simulink model "TST_CrCtl_Governor"  (R2016b)
settings: Solver=FixedStepDiscrete  StartTime=0.0  StopTime=simTime  FixedStep=sampleTime  RelTol=1e-3
values from neighbouring files (symbols this model uses):
  testCase = 1    [initTST_CrCtl_Governor_001.m]    (also in initTST_CrCtl_Governor_002.m = 2; initTST_CrCtl_Governor_003.m = 3; initTST_CrCtl_Governor_004.m = 4; initTST_CrCtl_Governor_005.m = 5)
libraries: simulink x144, UnitTest_Lib x110
(part 2 of 7)

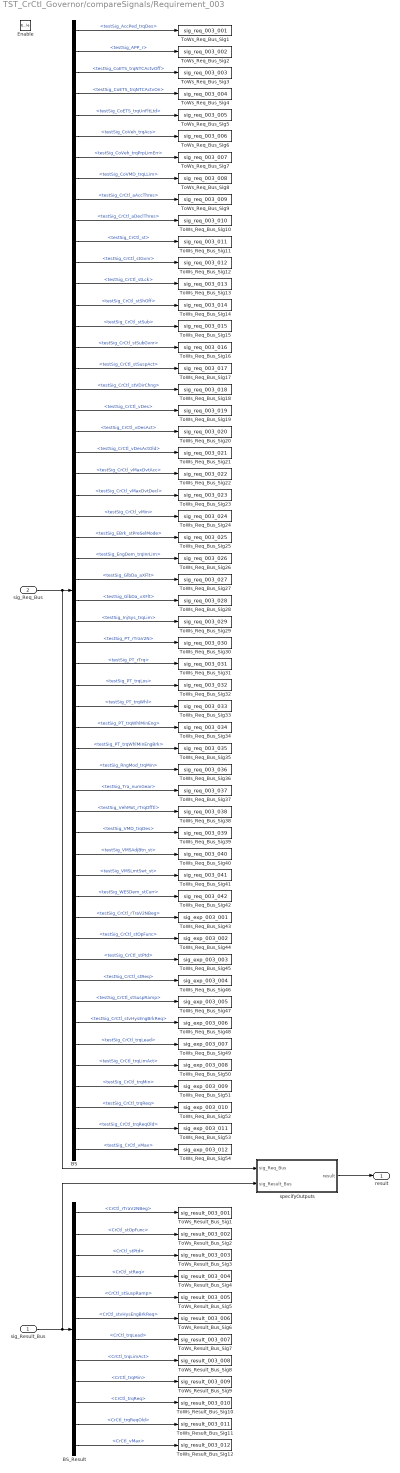
== system TST_CrCtl_Governor/compareSignals/Requirement_003 ==
  sig_Result_Bus : Inport
  sig_Req_Bus : Inport  Port=2
  Enable : EnablePort
  BS : BusSelector  OutputSignals=testSig_AccPed_trqDes,testSig_APP_r,testSig_CoETS_trqNTCActvOff,testSig_CoETS_trqNTCActvOn,testSig_CoETS_trqUnFltLtd,testSig_CoVeh_trqAcs,testSig_CoVeh_trqPrpLimErr,testSig_CoVMD_trqLLim,testSig_CrCtl_aAccThres,testSig_CrCtl_aDeclThres,testSig_CrCtl_st,testSig_CrCtl_stGvnr,testSig_CrCtl_stLck,testSig_CrCtl_stShOff,testSig_CrCtl_stSub,testSig_CrCtl_stSubGvnr,testSig_CrCtl_stSuspAct,testSig_CrCtl_stVDirChng,testSig_CrCtl_vDes,testSig_CrCtl_vDesAct,testSig_CrCtl_vDesActOld,testSig_CrCtl_vMaxDvtAcc,testSig_CrCtl_vMaxDvtDecl,testSig_CrCtl_vMin,testSig_EBrk_stPreSelMode,testSig_EngDem_trqInrLim,testSig_GlbDa_aXFlt,testSig_GlbDa_vXFlt,testSig_InjSys_trqLim,testSig_PT_rTraV2N,testSig_PT_rTrq,testSig_PT_trqLos,testSig_PT_trqWhl,testSig_PT_trqWhlMinEng,testSig_PT_trqWhlMinEngBrk,testSig_RngMod_trqMin,testSig_Tra_numGear,testSig_VehMot_rTrqDfftl,testSig_VMD_trqDes,testSig_VMSAdjBtn_st,testSig_VMSLmtSwt_st,testSig_WESDem_stCurr,testSig_CrCtl_rTraV2NBeg,testSig_CrCtl_stOpFunc,testSig_CrCtl_stPtd,testSig_CrCtl_stReq,testSig_CrCtl_stSuspRamp,testSig_CrCtl_stvHysEngBrkReq,testSig_CrCtl_trqLead,testSig_CrCtl_trqLimAct,testSig_CrCtl_trqMin,testSig_CrCtl_trqReq,testSig_CrCtl_trqReqOld,testSig_CrCtl_vMax
  BS_Result : BusSelector  OutputSignals=CrCtl_rTraV2NBeg,CrCtl_stOpFunc,CrCtl_stPtd,CrCtl_stReq,CrCtl_stSuspRamp,CrCtl_stvHysEngBrkReq,CrCtl_trqLead,CrCtl_trqLimAct,CrCtl_trqMin,CrCtl_trqReq,CrCtl_trqReqOld,CrCtl_vMax
  ToWs_Req_Bus_Sig1 : ToWorkspace  VariableName=sig_req_003_001  SaveFormat=Structure With Time
  ToWs_Req_Bus_Sig10 : ToWorkspace  VariableName=sig_req_003_010  SaveFormat=Structure With Time
  ToWs_Req_Bus_Sig11 : ToWorkspace  VariableName=sig_req_003_011  SaveFormat=Structure With Time
  ToWs_Req_Bus_Sig12 : ToWorkspace  VariableName=sig_req_003_012  SaveFormat=Structure With Time
  ToWs_Req_Bus_Sig13 : ToWorkspace  VariableName=sig_req_003_013  SaveFormat=Structure With Time
  ToWs_Req_Bus_Sig14 : ToWorkspace  VariableName=sig_req_003_014  SaveFormat=Structure With Time
  ToWs_Req_Bus_Sig15 : ToWorkspace  VariableName=sig_req_003_015  SaveFormat=Structure With Time
  ToWs_Req_Bus_Sig16 : ToWorkspace  VariableName=sig_req_003_016  SaveFormat=Structure With Time
  ToWs_Req_Bus_Sig17 : ToWorkspace  VariableName=sig_req_003_017  SaveFormat=Structure With Time
  ToWs_Req_Bus_Sig18 : ToWorkspace  VariableName=sig_req_003_018  SaveFormat=Structure With Time
  ToWs_Req_Bus_Sig19 : ToWorkspace  VariableName=sig_req_003_019  SaveFormat=Structure With Time
  ToWs_Req_Bus_Sig2 : ToWorkspace  VariableName=sig_req_003_002  SaveFormat=Structure With Time
  ToWs_Req_Bus_Sig20 : ToWorkspace  VariableName=sig_req_003_020  SaveFormat=Structure With Time
  ToWs_Req_Bus_Sig21 : ToWorkspace  VariableName=sig_req_003_021  SaveFormat=Structure With Time
  ToWs_Req_Bus_Sig22 : ToWorkspace  VariableName=sig_req_003_022  SaveFormat=Structure With Time
  ToWs_Req_Bus_Sig23 : ToWorkspace  VariableName=sig_req_003_023  SaveFormat=Structure With Time
  ToWs_Req_Bus_Sig24 : ToWorkspace  VariableName=sig_req_003_024  SaveFormat=Structure With Time
  ToWs_Req_Bus_Sig25 : ToWorkspace  VariableName=sig_req_003_025  SaveFormat=Structure With Time
  ToWs_Req_Bus_Sig26 : ToWorkspace  VariableName=sig_req_003_026  SaveFormat=Structure With Time
  ToWs_Req_Bus_Sig27 : ToWorkspace  VariableName=sig_req_003_027  SaveFormat=Structure With Time
  ToWs_Req_Bus_Sig28 : ToWorkspace  VariableName=sig_req_003_028  SaveFormat=Structure With Time
  ToWs_Req_Bus_Sig29 : ToWorkspace  VariableName=sig_req_003_029  SaveFormat=Structure With Time
  ToWs_Req_Bus_Sig3 : ToWorkspace  VariableName=sig_req_003_003  SaveFormat=Structure With Time
  ToWs_Req_Bus_Sig30 : ToWorkspace  VariableName=sig_req_003_030  SaveFormat=Structure With Time
  ToWs_Req_Bus_Sig31 : ToWorkspace  VariableName=sig_req_003_031  SaveFormat=Structure With Time
  ToWs_Req_Bus_Sig32 : ToWorkspace  VariableName=sig_req_003_032  SaveFormat=Structure With Time
  ToWs_Req_Bus_Sig33 : ToWorkspace  VariableName=sig_req_003_033  SaveFormat=Structure With Time
  ToWs_Req_Bus_Sig34 : ToWorkspace  VariableName=sig_req_003_034  SaveFormat=Structure With Time
  ToWs_Req_Bus_Sig35 : ToWorkspace  VariableName=sig_req_003_035  SaveFormat=Structure With Time
  ToWs_Req_Bus_Sig36 : ToWorkspace  VariableName=sig_req_003_036  SaveFormat=Structure With Time
  ToWs_Req_Bus_Sig37 : ToWorkspace  VariableName=sig_req_003_037  SaveFormat=Structure With Time
  ToWs_Req_Bus_Sig38 : ToWorkspace  VariableName=sig_req_003_038  SaveFormat=Structure With Time
  ToWs_Req_Bus_Sig39 : ToWorkspace  VariableName=sig_req_003_039  SaveFormat=Structure With Time
  ToWs_Req_Bus_Sig4 : ToWorkspace  VariableName=sig_req_003_004  SaveFormat=Structure With Time
  ToWs_Req_Bus_Sig40 : ToWorkspace  VariableName=sig_req_003_040  SaveFormat=Structure With Time
  ToWs_Req_Bus_Sig41 : ToWorkspace  VariableName=sig_req_003_041  SaveFormat=Structure With Time
  ToWs_Req_Bus_Sig42 : ToWorkspace  VariableName=sig_req_003_042  SaveFormat=Structure With Time
  ToWs_Req_Bus_Sig43 : ToWorkspace  VariableName=sig_exp_003_001  SaveFormat=Structure With Time
  ToWs_Req_Bus_Sig44 : ToWorkspace  VariableName=sig_exp_003_002  SaveFormat=Structure With Time
  ToWs_Req_Bus_Sig45 : ToWorkspace  VariableName=sig_exp_003_003  SaveFormat=Structure With Time
  ToWs_Req_Bus_Sig46 : ToWorkspace  VariableName=sig_exp_003_004  SaveFormat=Structure With Time
  ToWs_Req_Bus_Sig47 : ToWorkspace  VariableName=sig_exp_003_005  SaveFormat=Structure With Time
  ToWs_Req_Bus_Sig48 : ToWorkspace  VariableName=sig_exp_003_006  SaveFormat=Structure With Time
  ToWs_Req_Bus_Sig49 : ToWorkspace  VariableName=sig_exp_003_007  SaveFormat=Structure With Time
  ToWs_Req_Bus_Sig5 : ToWorkspace  VariableName=sig_req_003_005  SaveFormat=Structure With Time
  ToWs_Req_Bus_Sig50 : ToWorkspace  VariableName=sig_exp_003_008  SaveFormat=Structure With Time
  ToWs_Req_Bus_Sig51 : ToWorkspace  VariableName=sig_exp_003_009  SaveFormat=Structure With Time
  ToWs_Req_Bus_Sig52 : ToWorkspace  VariableName=sig_exp_003_010  SaveFormat=Structure With Time
  ToWs_Req_Bus_Sig53 : ToWorkspace  VariableName=sig_exp_003_011  SaveFormat=Structure With Time
  ToWs_Req_Bus_Sig54 : ToWorkspace  VariableName=sig_exp_003_012  SaveFormat=Structure With Time
  ToWs_Req_Bus_Sig6 : ToWorkspace  VariableName=sig_req_003_006  SaveFormat=Structure With Time
  ToWs_Req_Bus_Sig7 : ToWorkspace  VariableName=sig_req_003_007  SaveFormat=Structure With Time
  ToWs_Req_Bus_Sig8 : ToWorkspace  VariableName=sig_req_003_008  SaveFormat=Structure With Time
  ToWs_Req_Bus_Sig9 : ToWorkspace  VariableName=sig_req_003_009  SaveFormat=Structure With Time
  ToWs_Result_Bus_Sig1 : ToWorkspace  VariableName=sig_result_003_001  SaveFormat=Structure With Time
  ToWs_Result_Bus_Sig10 : ToWorkspace  VariableName=sig_result_003_010  SaveFormat=Structure With Time
  ToWs_Result_Bus_Sig11 : ToWorkspace  VariableName=sig_result_003_011  SaveFormat=Structure With Time
  ToWs_Result_Bus_Sig12 : ToWorkspace  VariableName=sig_result_003_012  SaveFormat=Structure With Time
  ToWs_Result_Bus_Sig2 : ToWorkspace  VariableName=sig_result_003_002  SaveFormat=Structure With Time
  ToWs_Result_Bus_Sig3 : ToWorkspace  VariableName=sig_result_003_003  SaveFormat=Structure With Time
  ToWs_Result_Bus_Sig4 : ToWorkspace  VariableName=sig_result_003_004  SaveFormat=Structure With Time
  ToWs_Result_Bus_Sig5 : ToWorkspace  VariableName=sig_result_003_005  SaveFormat=Structure With Time
  ToWs_Result_Bus_Sig6 : ToWorkspace  VariableName=sig_result_003_006  SaveFormat=Structure With Time
  ToWs_Result_Bus_Sig7 : ToWorkspace  VariableName=sig_result_003_007  SaveFormat=Structure With Time
  ToWs_Result_Bus_Sig8 : ToWorkspace  VariableName=sig_result_003_008  SaveFormat=Structure With Time
  ToWs_Result_Bus_Sig9 : ToWorkspace  VariableName=sig_result_003_009  SaveFormat=Structure With Time
  specifyOutputs : Subsystem
  result : Outport
  wires:
  sig_Req_Bus/1 -> BS/1, specifyOutputs/1(sig_Req_Bus)
  BS/1 -> ToWs_Req_Bus_Sig1/1  "<testSig_AccPed_trqDes>"
  BS/2 -> ToWs_Req_Bus_Sig2/1  "<testSig_APP_r>"
  BS/3 -> ToWs_Req_Bus_Sig3/1  "<testSig_CoETS_trqNTCActvOff>"
  BS/4 -> ToWs_Req_Bus_Sig4/1  "<testSig_CoETS_trqNTCActvOn>"
  BS/5 -> ToWs_Req_Bus_Sig5/1  "<testSig_CoETS_trqUnFltLtd>"
  BS/6 -> ToWs_Req_Bus_Sig6/1  "<testSig_CoVeh_trqAcs>"
  BS/7 -> ToWs_Req_Bus_Sig7/1  "<testSig_CoVeh_trqPrpLimErr>"
  BS/8 -> ToWs_Req_Bus_Sig8/1  "<testSig_CoVMD_trqLLim>"
  BS/9 -> ToWs_Req_Bus_Sig9/1  "<testSig_CrCtl_aAccThres>"
  BS/10 -> ToWs_Req_Bus_Sig10/1  "<testSig_CrCtl_aDeclThres>"
  BS/11 -> ToWs_Req_Bus_Sig11/1  "<testSig_CrCtl_st>"
  BS/12 -> ToWs_Req_Bus_Sig12/1  "<testSig_CrCtl_stGvnr>"
  BS/13 -> ToWs_Req_Bus_Sig13/1  "<testSig_CrCtl_stLck>"
  BS/14 -> ToWs_Req_Bus_Sig14/1  "<testSig_CrCtl_stShOff>"
  BS/15 -> ToWs_Req_Bus_Sig15/1  "<testSig_CrCtl_stSub>"
  BS/16 -> ToWs_Req_Bus_Sig16/1  "<testSig_CrCtl_stSubGvnr>"
  BS/17 -> ToWs_Req_Bus_Sig17/1  "<testSig_CrCtl_stSuspAct>"
  BS/18 -> ToWs_Req_Bus_Sig18/1  "<testSig_CrCtl_stVDirChng>"
  BS/19 -> ToWs_Req_Bus_Sig19/1  "<testSig_CrCtl_vDes>"
  BS/20 -> ToWs_Req_Bus_Sig20/1  "<testSig_CrCtl_vDesAct>"
  BS/21 -> ToWs_Req_Bus_Sig21/1  "<testSig_CrCtl_vDesActOld>"
  BS/22 -> ToWs_Req_Bus_Sig22/1  "<testSig_CrCtl_vMaxDvtAcc>"
  BS/23 -> ToWs_Req_Bus_Sig23/1  "<testSig_CrCtl_vMaxDvtDecl>"
  BS/24 -> ToWs_Req_Bus_Sig24/1  "<testSig_CrCtl_vMin>"
  BS/25 -> ToWs_Req_Bus_Sig25/1  "<testSig_EBrk_stPreSelMode>"
  BS/26 -> ToWs_Req_Bus_Sig26/1  "<testSig_EngDem_trqInrLim>"
  BS/27 -> ToWs_Req_Bus_Sig27/1  "<testSig_GlbDa_aXFlt>"
  BS/28 -> ToWs_Req_Bus_Sig28/1  "<testSig_GlbDa_vXFlt>"
  BS/29 -> ToWs_Req_Bus_Sig29/1  "<testSig_InjSys_trqLim>"
  BS/30 -> ToWs_Req_Bus_Sig30/1  "<testSig_PT_rTraV2N>"
  BS/31 -> ToWs_Req_Bus_Sig31/1  "<testSig_PT_rTrq>"
  BS/32 -> ToWs_Req_Bus_Sig32/1  "<testSig_PT_trqLos>"
  BS/33 -> ToWs_Req_Bus_Sig33/1  "<testSig_PT_trqWhl>"
  BS/34 -> ToWs_Req_Bus_Sig34/1  "<testSig_PT_trqWhlMinEng>"
  BS/35 -> ToWs_Req_Bus_Sig35/1  "<testSig_PT_trqWhlMinEngBrk>"
  BS/36 -> ToWs_Req_Bus_Sig36/1  "<testSig_RngMod_trqMin>"
  BS/37 -> ToWs_Req_Bus_Sig37/1  "<testSig_Tra_numGear>"
  BS/38 -> ToWs_Req_Bus_Sig38/1  "<testSig_VehMot_rTrqDfftl>"
  BS/39 -> ToWs_Req_Bus_Sig39/1  "<testSig_VMD_trqDes>"
  BS/40 -> ToWs_Req_Bus_Sig40/1  "<testSig_VMSAdjBtn_st>"
  BS/41 -> ToWs_Req_Bus_Sig41/1  "<testSig_VMSLmtSwt_st>"
  BS/42 -> ToWs_Req_Bus_Sig42/1  "<testSig_WESDem_stCurr>"
  BS/43 -> ToWs_Req_Bus_Sig43/1  "<testSig_CrCtl_rTraV2NBeg>"
  BS/44 -> ToWs_Req_Bus_Sig44/1  "<testSig_CrCtl_stOpFunc>"
  BS/45 -> ToWs_Req_Bus_Sig45/1  "<testSig_CrCtl_stPtd>"
  BS/46 -> ToWs_Req_Bus_Sig46/1  "<testSig_CrCtl_stReq>"
  BS/47 -> ToWs_Req_Bus_Sig47/1  "<testSig_CrCtl_stSuspRamp>"
  BS/48 -> ToWs_Req_Bus_Sig48/1  "<testSig_CrCtl_stvHysEngBrkReq>"
  BS/49 -> ToWs_Req_Bus_Sig49/1  "<testSig_CrCtl_trqLead>"
  BS/50 -> ToWs_Req_Bus_Sig50/1  "<testSig_CrCtl_trqLimAct>"
  BS/51 -> ToWs_Req_Bus_Sig51/1  "<testSig_CrCtl_trqMin>"
  BS/52 -> ToWs_Req_Bus_Sig52/1  "<testSig_CrCtl_trqReq>"
  BS/53 -> ToWs_Req_Bus_Sig53/1  "<testSig_CrCtl_trqReqOld>"
  BS/54 -> ToWs_Req_Bus_Sig54/1  "<testSig_CrCtl_vMax>"
  sig_Result_Bus/1 -> BS_Result/1, specifyOutputs/2(sig_Result_Bus)
  BS_Result/1 -> ToWs_Result_Bus_Sig1/1  "<CrCtl_rTraV2NBeg>"
  BS_Result/2 -> ToWs_Result_Bus_Sig2/1  "<CrCtl_stOpFunc>"
  BS_Result/3 -> ToWs_Result_Bus_Sig3/1  "<CrCtl_stPtd>"
  BS_Result/4 -> ToWs_Result_Bus_Sig4/1  "<CrCtl_stReq>"
  BS_Result/5 -> ToWs_Result_Bus_Sig5/1  "<CrCtl_stSuspRamp>"
  BS_Result/6 -> ToWs_Result_Bus_Sig6/1  "<CrCtl_stvHysEngBrkReq>"
  BS_Result/7 -> ToWs_Result_Bus_Sig7/1  "<CrCtl_trqLead>"
  BS_Result/8 -> ToWs_Result_Bus_Sig8/1  "<CrCtl_trqLimAct>"
  BS_Result/9 -> ToWs_Result_Bus_Sig9/1  "<CrCtl_trqMin>"
  BS_Result/10 -> ToWs_Result_Bus_Sig10/1  "<CrCtl_trqReq>"
  BS_Result/11 -> ToWs_Result_Bus_Sig11/1  "<CrCtl_trqReqOld>"
  BS_Result/12 -> ToWs_Result_Bus_Sig12/1  "<CrCtl_vMax>"
  specifyOutputs/1(result) -> result/1

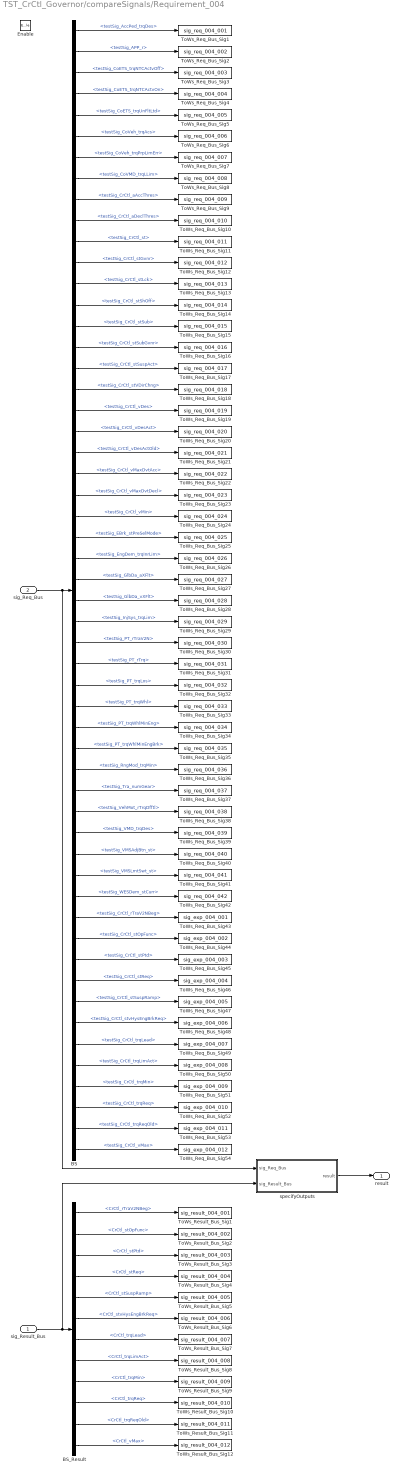
== system TST_CrCtl_Governor/compareSignals/Requirement_004 ==
  sig_Result_Bus : Inport
  sig_Req_Bus : Inport  Port=2
  Enable : EnablePort
  BS : BusSelector  OutputSignals=testSig_AccPed_trqDes,testSig_APP_r,testSig_CoETS_trqNTCActvOff,testSig_CoETS_trqNTCActvOn,testSig_CoETS_trqUnFltLtd,testSig_CoVeh_trqAcs,testSig_CoVeh_trqPrpLimErr,testSig_CoVMD_trqLLim,testSig_CrCtl_aAccThres,testSig_CrCtl_aDeclThres,testSig_CrCtl_st,testSig_CrCtl_stGvnr,testSig_CrCtl_stLck,testSig_CrCtl_stShOff,testSig_CrCtl_stSub,testSig_CrCtl_stSubGvnr,testSig_CrCtl_stSuspAct,testSig_CrCtl_stVDirChng,testSig_CrCtl_vDes,testSig_CrCtl_vDesAct,testSig_CrCtl_vDesActOld,testSig_CrCtl_vMaxDvtAcc,testSig_CrCtl_vMaxDvtDecl,testSig_CrCtl_vMin,testSig_EBrk_stPreSelMode,testSig_EngDem_trqInrLim,testSig_GlbDa_aXFlt,testSig_GlbDa_vXFlt,testSig_InjSys_trqLim,testSig_PT_rTraV2N,testSig_PT_rTrq,testSig_PT_trqLos,testSig_PT_trqWhl,testSig_PT_trqWhlMinEng,testSig_PT_trqWhlMinEngBrk,testSig_RngMod_trqMin,testSig_Tra_numGear,testSig_VehMot_rTrqDfftl,testSig_VMD_trqDes,testSig_VMSAdjBtn_st,testSig_VMSLmtSwt_st,testSig_WESDem_stCurr,testSig_CrCtl_rTraV2NBeg,testSig_CrCtl_stOpFunc,testSig_CrCtl_stPtd,testSig_CrCtl_stReq,testSig_CrCtl_stSuspRamp,testSig_CrCtl_stvHysEngBrkReq,testSig_CrCtl_trqLead,testSig_CrCtl_trqLimAct,testSig_CrCtl_trqMin,testSig_CrCtl_trqReq,testSig_CrCtl_trqReqOld,testSig_CrCtl_vMax
  BS_Result : BusSelector  OutputSignals=CrCtl_rTraV2NBeg,CrCtl_stOpFunc,CrCtl_stPtd,CrCtl_stReq,CrCtl_stSuspRamp,CrCtl_stvHysEngBrkReq,CrCtl_trqLead,CrCtl_trqLimAct,CrCtl_trqMin,CrCtl_trqReq,CrCtl_trqReqOld,CrCtl_vMax
  ToWs_Req_Bus_Sig1 : ToWorkspace  VariableName=sig_req_004_001  SaveFormat=Structure With Time
  ToWs_Req_Bus_Sig10 : ToWorkspace  VariableName=sig_req_004_010  SaveFormat=Structure With Time
  ToWs_Req_Bus_Sig11 : ToWorkspace  VariableName=sig_req_004_011  SaveFormat=Structure With Time
  ToWs_Req_Bus_Sig12 : ToWorkspace  VariableName=sig_req_004_012  SaveFormat=Structure With Time
  ToWs_Req_Bus_Sig13 : ToWorkspace  VariableName=sig_req_004_013  SaveFormat=Structure With Time
  ToWs_Req_Bus_Sig14 : ToWorkspace  VariableName=sig_req_004_014  SaveFormat=Structure With Time
  ToWs_Req_Bus_Sig15 : ToWorkspace  VariableName=sig_req_004_015  SaveFormat=Structure With Time
  ToWs_Req_Bus_Sig16 : ToWorkspace  VariableName=sig_req_004_016  SaveFormat=Structure With Time
  ToWs_Req_Bus_Sig17 : ToWorkspace  VariableName=sig_req_004_017  SaveFormat=Structure With Time
  ToWs_Req_Bus_Sig18 : ToWorkspace  VariableName=sig_req_004_018  SaveFormat=Structure With Time
  ToWs_Req_Bus_Sig19 : ToWorkspace  VariableName=sig_req_004_019  SaveFormat=Structure With Time
  ToWs_Req_Bus_Sig2 : ToWorkspace  VariableName=sig_req_004_002  SaveFormat=Structure With Time
  ToWs_Req_Bus_Sig20 : ToWorkspace  VariableName=sig_req_004_020  SaveFormat=Structure With Time
  ToWs_Req_Bus_Sig21 : ToWorkspace  VariableName=sig_req_004_021  SaveFormat=Structure With Time
  ToWs_Req_Bus_Sig22 : ToWorkspace  VariableName=sig_req_004_022  SaveFormat=Structure With Time
  ToWs_Req_Bus_Sig23 : ToWorkspace  VariableName=sig_req_004_023  SaveFormat=Structure With Time
  ToWs_Req_Bus_Sig24 : ToWorkspace  VariableName=sig_req_004_024  SaveFormat=Structure With Time
  ToWs_Req_Bus_Sig25 : ToWorkspace  VariableName=sig_req_004_025  SaveFormat=Structure With Time
  ToWs_Req_Bus_Sig26 : ToWorkspace  VariableName=sig_req_004_026  SaveFormat=Structure With Time
  ToWs_Req_Bus_Sig27 : ToWorkspace  VariableName=sig_req_004_027  SaveFormat=Structure With Time
  ToWs_Req_Bus_Sig28 : ToWorkspace  VariableName=sig_req_004_028  SaveFormat=Structure With Time
  ToWs_Req_Bus_Sig29 : ToWorkspace  VariableName=sig_req_004_029  SaveFormat=Structure With Time
  ToWs_Req_Bus_Sig3 : ToWorkspace  VariableName=sig_req_004_003  SaveFormat=Structure With Time
  ToWs_Req_Bus_Sig30 : ToWorkspace  VariableName=sig_req_004_030  SaveFormat=Structure With Time
  ToWs_Req_Bus_Sig31 : ToWorkspace  VariableName=sig_req_004_031  SaveFormat=Structure With Time
  ToWs_Req_Bus_Sig32 : ToWorkspace  VariableName=sig_req_004_032  SaveFormat=Structure With Time
  ToWs_Req_Bus_Sig33 : ToWorkspace  VariableName=sig_req_004_033  SaveFormat=Structure With Time
  ToWs_Req_Bus_Sig34 : ToWorkspace  VariableName=sig_req_004_034  SaveFormat=Structure With Time
  ToWs_Req_Bus_Sig35 : ToWorkspace  VariableName=sig_req_004_035  SaveFormat=Structure With Time
  ToWs_Req_Bus_Sig36 : ToWorkspace  VariableName=sig_req_004_036  SaveFormat=Structure With Time
  ToWs_Req_Bus_Sig37 : ToWorkspace  VariableName=sig_req_004_037  SaveFormat=Structure With Time
  ToWs_Req_Bus_Sig38 : ToWorkspace  VariableName=sig_req_004_038  SaveFormat=Structure With Time
  ToWs_Req_Bus_Sig39 : ToWorkspace  VariableName=sig_req_004_039  SaveFormat=Structure With Time
  ToWs_Req_Bus_Sig4 : ToWorkspace  VariableName=sig_req_004_004  SaveFormat=Structure With Time
  ToWs_Req_Bus_Sig40 : ToWorkspace  VariableName=sig_req_004_040  SaveFormat=Structure With Time
  ToWs_Req_Bus_Sig41 : ToWorkspace  VariableName=sig_req_004_041  SaveFormat=Structure With Time
  ToWs_Req_Bus_Sig42 : ToWorkspace  VariableName=sig_req_004_042  SaveFormat=Structure With Time
  ToWs_Req_Bus_Sig43 : ToWorkspace  VariableName=sig_exp_004_001  SaveFormat=Structure With Time
  ToWs_Req_Bus_Sig44 : ToWorkspace  VariableName=sig_exp_004_002  SaveFormat=Structure With Time
  ToWs_Req_Bus_Sig45 : ToWorkspace  VariableName=sig_exp_004_003  SaveFormat=Structure With Time
  ToWs_Req_Bus_Sig46 : ToWorkspace  VariableName=sig_exp_004_004  SaveFormat=Structure With Time
  ToWs_Req_Bus_Sig47 : ToWorkspace  VariableName=sig_exp_004_005  SaveFormat=Structure With Time
  ToWs_Req_Bus_Sig48 : ToWorkspace  VariableName=sig_exp_004_006  SaveFormat=Structure With Time
  ToWs_Req_Bus_Sig49 : ToWorkspace  VariableName=sig_exp_004_007  SaveFormat=Structure With Time
  ToWs_Req_Bus_Sig5 : ToWorkspace  VariableName=sig_req_004_005  SaveFormat=Structure With Time
  ToWs_Req_Bus_Sig50 : ToWorkspace  VariableName=sig_exp_004_008  SaveFormat=Structure With Time
  ToWs_Req_Bus_Sig51 : ToWorkspace  VariableName=sig_exp_004_009  SaveFormat=Structure With Time
  ToWs_Req_Bus_Sig52 : ToWorkspace  VariableName=sig_exp_004_010  SaveFormat=Structure With Time
  ToWs_Req_Bus_Sig53 : ToWorkspace  VariableName=sig_exp_004_011  SaveFormat=Structure With Time
  ToWs_Req_Bus_Sig54 : ToWorkspace  VariableName=sig_exp_004_012  SaveFormat=Structure With Time
  ToWs_Req_Bus_Sig6 : ToWorkspace  VariableName=sig_req_004_006  SaveFormat=Structure With Time
  ToWs_Req_Bus_Sig7 : ToWorkspace  VariableName=sig_req_004_007  SaveFormat=Structure With Time
  ToWs_Req_Bus_Sig8 : ToWorkspace  VariableName=sig_req_004_008  SaveFormat=Structure With Time
  ToWs_Req_Bus_Sig9 : ToWorkspace  VariableName=sig_req_004_009  SaveFormat=Structure With Time
  ToWs_Result_Bus_Sig1 : ToWorkspace  VariableName=sig_result_004_001  SaveFormat=Structure With Time
  ToWs_Result_Bus_Sig10 : ToWorkspace  VariableName=sig_result_004_010  SaveFormat=Structure With Time
  ToWs_Result_Bus_Sig11 : ToWorkspace  VariableName=sig_result_004_011  SaveFormat=Structure With Time
  ToWs_Result_Bus_Sig12 : ToWorkspace  VariableName=sig_result_004_012  SaveFormat=Structure With Time
  ToWs_Result_Bus_Sig2 : ToWorkspace  VariableName=sig_result_004_002  SaveFormat=Structure With Time
  ToWs_Result_Bus_Sig3 : ToWorkspace  VariableName=sig_result_004_003  SaveFormat=Structure With Time
  ToWs_Result_Bus_Sig4 : ToWorkspace  VariableName=sig_result_004_004  SaveFormat=Structure With Time
  ToWs_Result_Bus_Sig5 : ToWorkspace  VariableName=sig_result_004_005  SaveFormat=Structure With Time
  ToWs_Result_Bus_Sig6 : ToWorkspace  VariableName=sig_result_004_006  SaveFormat=Structure With Time
  ToWs_Result_Bus_Sig7 : ToWorkspace  VariableName=sig_result_004_007  SaveFormat=Structure With Time
  ToWs_Result_Bus_Sig8 : ToWorkspace  VariableName=sig_result_004_008  SaveFormat=Structure With Time
  ToWs_Result_Bus_Sig9 : ToWorkspace  VariableName=sig_result_004_009  SaveFormat=Structure With Time
  specifyOutputs : Subsystem
  result : Outport
  wires:
  sig_Req_Bus/1 -> BS/1, specifyOutputs/1(sig_Req_Bus)
  BS/1 -> ToWs_Req_Bus_Sig1/1  "<testSig_AccPed_trqDes>"
  BS/2 -> ToWs_Req_Bus_Sig2/1  "<testSig_APP_r>"
  BS/3 -> ToWs_Req_Bus_Sig3/1  "<testSig_CoETS_trqNTCActvOff>"
  BS/4 -> ToWs_Req_Bus_Sig4/1  "<testSig_CoETS_trqNTCActvOn>"
  BS/5 -> ToWs_Req_Bus_Sig5/1  "<testSig_CoETS_trqUnFltLtd>"
  BS/6 -> ToWs_Req_Bus_Sig6/1  "<testSig_CoVeh_trqAcs>"
  BS/7 -> ToWs_Req_Bus_Sig7/1  "<testSig_CoVeh_trqPrpLimErr>"
  BS/8 -> ToWs_Req_Bus_Sig8/1  "<testSig_CoVMD_trqLLim>"
  BS/9 -> ToWs_Req_Bus_Sig9/1  "<testSig_CrCtl_aAccThres>"
  BS/10 -> ToWs_Req_Bus_Sig10/1  "<testSig_CrCtl_aDeclThres>"
  BS/11 -> ToWs_Req_Bus_Sig11/1  "<testSig_CrCtl_st>"
  BS/12 -> ToWs_Req_Bus_Sig12/1  "<testSig_CrCtl_stGvnr>"
  BS/13 -> ToWs_Req_Bus_Sig13/1  "<testSig_CrCtl_stLck>"
  BS/14 -> ToWs_Req_Bus_Sig14/1  "<testSig_CrCtl_stShOff>"
  BS/15 -> ToWs_Req_Bus_Sig15/1  "<testSig_CrCtl_stSub>"
  BS/16 -> ToWs_Req_Bus_Sig16/1  "<testSig_CrCtl_stSubGvnr>"
  BS/17 -> ToWs_Req_Bus_Sig17/1  "<testSig_CrCtl_stSuspAct>"
  BS/18 -> ToWs_Req_Bus_Sig18/1  "<testSig_CrCtl_stVDirChng>"
  BS/19 -> ToWs_Req_Bus_Sig19/1  "<testSig_CrCtl_vDes>"
  BS/20 -> ToWs_Req_Bus_Sig20/1  "<testSig_CrCtl_vDesAct>"
  BS/21 -> ToWs_Req_Bus_Sig21/1  "<testSig_CrCtl_vDesActOld>"
  BS/22 -> ToWs_Req_Bus_Sig22/1  "<testSig_CrCtl_vMaxDvtAcc>"
  BS/23 -> ToWs_Req_Bus_Sig23/1  "<testSig_CrCtl_vMaxDvtDecl>"
  BS/24 -> ToWs_Req_Bus_Sig24/1  "<testSig_CrCtl_vMin>"
  BS/25 -> ToWs_Req_Bus_Sig25/1  "<testSig_EBrk_stPreSelMode>"
  BS/26 -> ToWs_Req_Bus_Sig26/1  "<testSig_EngDem_trqInrLim>"
  BS/27 -> ToWs_Req_Bus_Sig27/1  "<testSig_GlbDa_aXFlt>"
  BS/28 -> ToWs_Req_Bus_Sig28/1  "<testSig_GlbDa_vXFlt>"
  BS/29 -> ToWs_Req_Bus_Sig29/1  "<testSig_InjSys_trqLim>"
  BS/30 -> ToWs_Req_Bus_Sig30/1  "<testSig_PT_rTraV2N>"
  BS/31 -> ToWs_Req_Bus_Sig31/1  "<testSig_PT_rTrq>"
  BS/32 -> ToWs_Req_Bus_Sig32/1  "<testSig_PT_trqLos>"
  BS/33 -> ToWs_Req_Bus_Sig33/1  "<testSig_PT_trqWhl>"
  BS/34 -> ToWs_Req_Bus_Sig34/1  "<testSig_PT_trqWhlMinEng>"
  BS/35 -> ToWs_Req_Bus_Sig35/1  "<testSig_PT_trqWhlMinEngBrk>"
  BS/36 -> ToWs_Req_Bus_Sig36/1  "<testSig_RngMod_trqMin>"
  BS/37 -> ToWs_Req_Bus_Sig37/1  "<testSig_Tra_numGear>"
  BS/38 -> ToWs_Req_Bus_Sig38/1  "<testSig_VehMot_rTrqDfftl>"
  BS/39 -> ToWs_Req_Bus_Sig39/1  "<testSig_VMD_trqDes>"
  BS/40 -> ToWs_Req_Bus_Sig40/1  "<testSig_VMSAdjBtn_st>"
  BS/41 -> ToWs_Req_Bus_Sig41/1  "<testSig_VMSLmtSwt_st>"
  BS/42 -> ToWs_Req_Bus_Sig42/1  "<testSig_WESDem_stCurr>"
  BS/43 -> ToWs_Req_Bus_Sig43/1  "<testSig_CrCtl_rTraV2NBeg>"
  BS/44 -> ToWs_Req_Bus_Sig44/1  "<testSig_CrCtl_stOpFunc>"
  BS/45 -> ToWs_Req_Bus_Sig45/1  "<testSig_CrCtl_stPtd>"
  BS/46 -> ToWs_Req_Bus_Sig46/1  "<testSig_CrCtl_stReq>"
  BS/47 -> ToWs_Req_Bus_Sig47/1  "<testSig_CrCtl_stSuspRamp>"
  BS/48 -> ToWs_Req_Bus_Sig48/1  "<testSig_CrCtl_stvHysEngBrkReq>"
  BS/49 -> ToWs_Req_Bus_Sig49/1  "<testSig_CrCtl_trqLead>"
  BS/50 -> ToWs_Req_Bus_Sig50/1  "<testSig_CrCtl_trqLimAct>"
  BS/51 -> ToWs_Req_Bus_Sig51/1  "<testSig_CrCtl_trqMin>"
  BS/52 -> ToWs_Req_Bus_Sig52/1  "<testSig_CrCtl_trqReq>"
  BS/53 -> ToWs_Req_Bus_Sig53/1  "<testSig_CrCtl_trqReqOld>"
  BS/54 -> ToWs_Req_Bus_Sig54/1  "<testSig_CrCtl_vMax>"
  sig_Result_Bus/1 -> BS_Result/1, specifyOutputs/2(sig_Result_Bus)
  BS_Result/1 -> ToWs_Result_Bus_Sig1/1  "<CrCtl_rTraV2NBeg>"
  BS_Result/2 -> ToWs_Result_Bus_Sig2/1  "<CrCtl_stOpFunc>"
  BS_Result/3 -> ToWs_Result_Bus_Sig3/1  "<CrCtl_stPtd>"
  BS_Result/4 -> ToWs_Result_Bus_Sig4/1  "<CrCtl_stReq>"
  BS_Result/5 -> ToWs_Result_Bus_Sig5/1  "<CrCtl_stSuspRamp>"
  BS_Result/6 -> ToWs_Result_Bus_Sig6/1  "<CrCtl_stvHysEngBrkReq>"
  BS_Result/7 -> ToWs_Result_Bus_Sig7/1  "<CrCtl_trqLead>"
  BS_Result/8 -> ToWs_Result_Bus_Sig8/1  "<CrCtl_trqLimAct>"
  BS_Result/9 -> ToWs_Result_Bus_Sig9/1  "<CrCtl_trqMin>"
  BS_Result/10 -> ToWs_Result_Bus_Sig10/1  "<CrCtl_trqReq>"
  BS_Result/11 -> ToWs_Result_Bus_Sig11/1  "<CrCtl_trqReqOld>"
  BS_Result/12 -> ToWs_Result_Bus_Sig12/1  "<CrCtl_vMax>"
  specifyOutputs/1(result) -> result/1

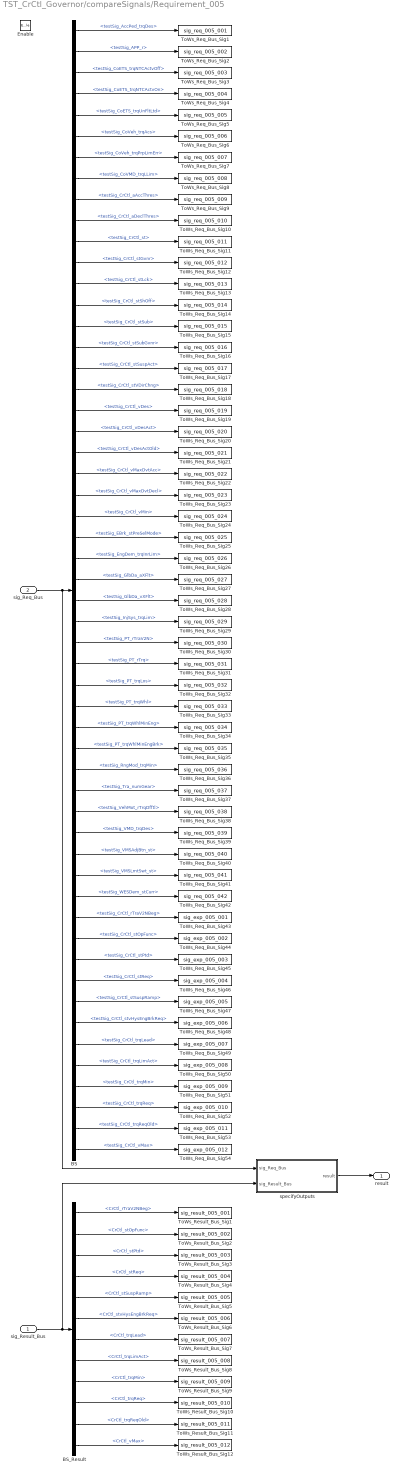
== system TST_CrCtl_Governor/compareSignals/Requirement_005 ==
  sig_Result_Bus : Inport
  sig_Req_Bus : Inport  Port=2
  Enable : EnablePort
  BS : BusSelector  OutputSignals=testSig_AccPed_trqDes,testSig_APP_r,testSig_CoETS_trqNTCActvOff,testSig_CoETS_trqNTCActvOn,testSig_CoETS_trqUnFltLtd,testSig_CoVeh_trqAcs,testSig_CoVeh_trqPrpLimErr,testSig_CoVMD_trqLLim,testSig_CrCtl_aAccThres,testSig_CrCtl_aDeclThres,testSig_CrCtl_st,testSig_CrCtl_stGvnr,testSig_CrCtl_stLck,testSig_CrCtl_stShOff,testSig_CrCtl_stSub,testSig_CrCtl_stSubGvnr,testSig_CrCtl_stSuspAct,testSig_CrCtl_stVDirChng,testSig_CrCtl_vDes,testSig_CrCtl_vDesAct,testSig_CrCtl_vDesActOld,testSig_CrCtl_vMaxDvtAcc,testSig_CrCtl_vMaxDvtDecl,testSig_CrCtl_vMin,testSig_EBrk_stPreSelMode,testSig_EngDem_trqInrLim,testSig_GlbDa_aXFlt,testSig_GlbDa_vXFlt,testSig_InjSys_trqLim,testSig_PT_rTraV2N,testSig_PT_rTrq,testSig_PT_trqLos,testSig_PT_trqWhl,testSig_PT_trqWhlMinEng,testSig_PT_trqWhlMinEngBrk,testSig_RngMod_trqMin,testSig_Tra_numGear,testSig_VehMot_rTrqDfftl,testSig_VMD_trqDes,testSig_VMSAdjBtn_st,testSig_VMSLmtSwt_st,testSig_WESDem_stCurr,testSig_CrCtl_rTraV2NBeg,testSig_CrCtl_stOpFunc,testSig_CrCtl_stPtd,testSig_CrCtl_stReq,testSig_CrCtl_stSuspRamp,testSig_CrCtl_stvHysEngBrkReq,testSig_CrCtl_trqLead,testSig_CrCtl_trqLimAct,testSig_CrCtl_trqMin,testSig_CrCtl_trqReq,testSig_CrCtl_trqReqOld,testSig_CrCtl_vMax
  BS_Result : BusSelector  OutputSignals=CrCtl_rTraV2NBeg,CrCtl_stOpFunc,CrCtl_stPtd,CrCtl_stReq,CrCtl_stSuspRamp,CrCtl_stvHysEngBrkReq,CrCtl_trqLead,CrCtl_trqLimAct,CrCtl_trqMin,CrCtl_trqReq,CrCtl_trqReqOld,CrCtl_vMax
  ToWs_Req_Bus_Sig1 : ToWorkspace  VariableName=sig_req_005_001  SaveFormat=Structure With Time
  ToWs_Req_Bus_Sig10 : ToWorkspace  VariableName=sig_req_005_010  SaveFormat=Structure With Time
  ToWs_Req_Bus_Sig11 : ToWorkspace  VariableName=sig_req_005_011  SaveFormat=Structure With Time
  ToWs_Req_Bus_Sig12 : ToWorkspace  VariableName=sig_req_005_012  SaveFormat=Structure With Time
  ToWs_Req_Bus_Sig13 : ToWorkspace  VariableName=sig_req_005_013  SaveFormat=Structure With Time
  ToWs_Req_Bus_Sig14 : ToWorkspace  VariableName=sig_req_005_014  SaveFormat=Structure With Time
  ToWs_Req_Bus_Sig15 : ToWorkspace  VariableName=sig_req_005_015  SaveFormat=Structure With Time
  ToWs_Req_Bus_Sig16 : ToWorkspace  VariableName=sig_req_005_016  SaveFormat=Structure With Time
  ToWs_Req_Bus_Sig17 : ToWorkspace  VariableName=sig_req_005_017  SaveFormat=Structure With Time
  ToWs_Req_Bus_Sig18 : ToWorkspace  VariableName=sig_req_005_018  SaveFormat=Structure With Time
  ToWs_Req_Bus_Sig19 : ToWorkspace  VariableName=sig_req_005_019  SaveFormat=Structure With Time
  ToWs_Req_Bus_Sig2 : ToWorkspace  VariableName=sig_req_005_002  SaveFormat=Structure With Time
  ToWs_Req_Bus_Sig20 : ToWorkspace  VariableName=sig_req_005_020  SaveFormat=Structure With Time
  ToWs_Req_Bus_Sig21 : ToWorkspace  VariableName=sig_req_005_021  SaveFormat=Structure With Time
  ToWs_Req_Bus_Sig22 : ToWorkspace  VariableName=sig_req_005_022  SaveFormat=Structure With Time
  ToWs_Req_Bus_Sig23 : ToWorkspace  VariableName=sig_req_005_023  SaveFormat=Structure With Time
  ToWs_Req_Bus_Sig24 : ToWorkspace  VariableName=sig_req_005_024  SaveFormat=Structure With Time
  ToWs_Req_Bus_Sig25 : ToWorkspace  VariableName=sig_req_005_025  SaveFormat=Structure With Time
  ToWs_Req_Bus_Sig26 : ToWorkspace  VariableName=sig_req_005_026  SaveFormat=Structure With Time
  ToWs_Req_Bus_Sig27 : ToWorkspace  VariableName=sig_req_005_027  SaveFormat=Structure With Time
  ToWs_Req_Bus_Sig28 : ToWorkspace  VariableName=sig_req_005_028  SaveFormat=Structure With Time
  ToWs_Req_Bus_Sig29 : ToWorkspace  VariableName=sig_req_005_029  SaveFormat=Structure With Time
  ToWs_Req_Bus_Sig3 : ToWorkspace  VariableName=sig_req_005_003  SaveFormat=Structure With Time
  ToWs_Req_Bus_Sig30 : ToWorkspace  VariableName=sig_req_005_030  SaveFormat=Structure With Time
  ToWs_Req_Bus_Sig31 : ToWorkspace  VariableName=sig_req_005_031  SaveFormat=Structure With Time
  ToWs_Req_Bus_Sig32 : ToWorkspace  VariableName=sig_req_005_032  SaveFormat=Structure With Time
  ToWs_Req_Bus_Sig33 : ToWorkspace  VariableName=sig_req_005_033  SaveFormat=Structure With Time
  ToWs_Req_Bus_Sig34 : ToWorkspace  VariableName=sig_req_005_034  SaveFormat=Structure With Time
  ToWs_Req_Bus_Sig35 : ToWorkspace  VariableName=sig_req_005_035  SaveFormat=Structure With Time
  ToWs_Req_Bus_Sig36 : ToWorkspace  VariableName=sig_req_005_036  SaveFormat=Structure With Time
  ToWs_Req_Bus_Sig37 : ToWorkspace  VariableName=sig_req_005_037  SaveFormat=Structure With Time
  ToWs_Req_Bus_Sig38 : ToWorkspace  VariableName=sig_req_005_038  SaveFormat=Structure With Time
  ToWs_Req_Bus_Sig39 : ToWorkspace  VariableName=sig_req_005_039  SaveFormat=Structure With Time
  ToWs_Req_Bus_Sig4 : ToWorkspace  VariableName=sig_req_005_004  SaveFormat=Structure With Time
  ToWs_Req_Bus_Sig40 : ToWorkspace  VariableName=sig_req_005_040  SaveFormat=Structure With Time
  ToWs_Req_Bus_Sig41 : ToWorkspace  VariableName=sig_req_005_041  SaveFormat=Structure With Time
  ToWs_Req_Bus_Sig42 : ToWorkspace  VariableName=sig_req_005_042  SaveFormat=Structure With Time
  ToWs_Req_Bus_Sig43 : ToWorkspace  VariableName=sig_exp_005_001  SaveFormat=Structure With Time
  ToWs_Req_Bus_Sig44 : ToWorkspace  VariableName=sig_exp_005_002  SaveFormat=Structure With Time
  ToWs_Req_Bus_Sig45 : ToWorkspace  VariableName=sig_exp_005_003  SaveFormat=Structure With Time
  ToWs_Req_Bus_Sig46 : ToWorkspace  VariableName=sig_exp_005_004  SaveFormat=Structure With Time
  ToWs_Req_Bus_Sig47 : ToWorkspace  VariableName=sig_exp_005_005  SaveFormat=Structure With Time
  ToWs_Req_Bus_Sig48 : ToWorkspace  VariableName=sig_exp_005_006  SaveFormat=Structure With Time
  ToWs_Req_Bus_Sig49 : ToWorkspace  VariableName=sig_exp_005_007  SaveFormat=Structure With Time
  ToWs_Req_Bus_Sig5 : ToWorkspace  VariableName=sig_req_005_005  SaveFormat=Structure With Time
  ToWs_Req_Bus_Sig50 : ToWorkspace  VariableName=sig_exp_005_008  SaveFormat=Structure With Time
  ToWs_Req_Bus_Sig51 : ToWorkspace  VariableName=sig_exp_005_009  SaveFormat=Structure With Time
  ToWs_Req_Bus_Sig52 : ToWorkspace  VariableName=sig_exp_005_010  SaveFormat=Structure With Time
  ToWs_Req_Bus_Sig53 : ToWorkspace  VariableName=sig_exp_005_011  SaveFormat=Structure With Time
  ToWs_Req_Bus_Sig54 : ToWorkspace  VariableName=sig_exp_005_012  SaveFormat=Structure With Time
  ToWs_Req_Bus_Sig6 : ToWorkspace  VariableName=sig_req_005_006  SaveFormat=Structure With Time
  ToWs_Req_Bus_Sig7 : ToWorkspace  VariableName=sig_req_005_007  SaveFormat=Structure With Time
  ToWs_Req_Bus_Sig8 : ToWorkspace  VariableName=sig_req_005_008  SaveFormat=Structure With Time
  ToWs_Req_Bus_Sig9 : ToWorkspace  VariableName=sig_req_005_009  SaveFormat=Structure With Time
  ToWs_Result_Bus_Sig1 : ToWorkspace  VariableName=sig_result_005_001  SaveFormat=Structure With Time
  ToWs_Result_Bus_Sig10 : ToWorkspace  VariableName=sig_result_005_010  SaveFormat=Structure With Time
  ToWs_Result_Bus_Sig11 : ToWorkspace  VariableName=sig_result_005_011  SaveFormat=Structure With Time
  ToWs_Result_Bus_Sig12 : ToWorkspace  VariableName=sig_result_005_012  SaveFormat=Structure With Time
  ToWs_Result_Bus_Sig2 : ToWorkspace  VariableName=sig_result_005_002  SaveFormat=Structure With Time
  ToWs_Result_Bus_Sig3 : ToWorkspace  VariableName=sig_result_005_003  SaveFormat=Structure With Time
  ToWs_Result_Bus_Sig4 : ToWorkspace  VariableName=sig_result_005_004  SaveFormat=Structure With Time
  ToWs_Result_Bus_Sig5 : ToWorkspace  VariableName=sig_result_005_005  SaveFormat=Structure With Time
  ToWs_Result_Bus_Sig6 : ToWorkspace  VariableName=sig_result_005_006  SaveFormat=Structure With Time
  ToWs_Result_Bus_Sig7 : ToWorkspace  VariableName=sig_result_005_007  SaveFormat=Structure With Time
  ToWs_Result_Bus_Sig8 : ToWorkspace  VariableName=sig_result_005_008  SaveFormat=Structure With Time
  ToWs_Result_Bus_Sig9 : ToWorkspace  VariableName=sig_result_005_009  SaveFormat=Structure With Time
  specifyOutputs : Subsystem
  result : Outport
  wires:
  sig_Req_Bus/1 -> BS/1, specifyOutputs/1(sig_Req_Bus)
  BS/1 -> ToWs_Req_Bus_Sig1/1  "<testSig_AccPed_trqDes>"
  BS/2 -> ToWs_Req_Bus_Sig2/1  "<testSig_APP_r>"
  BS/3 -> ToWs_Req_Bus_Sig3/1  "<testSig_CoETS_trqNTCActvOff>"
  BS/4 -> ToWs_Req_Bus_Sig4/1  "<testSig_CoETS_trqNTCActvOn>"
  BS/5 -> ToWs_Req_Bus_Sig5/1  "<testSig_CoETS_trqUnFltLtd>"
  BS/6 -> ToWs_Req_Bus_Sig6/1  "<testSig_CoVeh_trqAcs>"
  BS/7 -> ToWs_Req_Bus_Sig7/1  "<testSig_CoVeh_trqPrpLimErr>"
  BS/8 -> ToWs_Req_Bus_Sig8/1  "<testSig_CoVMD_trqLLim>"
  BS/9 -> ToWs_Req_Bus_Sig9/1  "<testSig_CrCtl_aAccThres>"
  BS/10 -> ToWs_Req_Bus_Sig10/1  "<testSig_CrCtl_aDeclThres>"
  BS/11 -> ToWs_Req_Bus_Sig11/1  "<testSig_CrCtl_st>"
  BS/12 -> ToWs_Req_Bus_Sig12/1  "<testSig_CrCtl_stGvnr>"
  BS/13 -> ToWs_Req_Bus_Sig13/1  "<testSig_CrCtl_stLck>"
  BS/14 -> ToWs_Req_Bus_Sig14/1  "<testSig_CrCtl_stShOff>"
  BS/15 -> ToWs_Req_Bus_Sig15/1  "<testSig_CrCtl_stSub>"
  BS/16 -> ToWs_Req_Bus_Sig16/1  "<testSig_CrCtl_stSubGvnr>"
  BS/17 -> ToWs_Req_Bus_Sig17/1  "<testSig_CrCtl_stSuspAct>"
  BS/18 -> ToWs_Req_Bus_Sig18/1  "<testSig_CrCtl_stVDirChng>"
  BS/19 -> ToWs_Req_Bus_Sig19/1  "<testSig_CrCtl_vDes>"
  BS/20 -> ToWs_Req_Bus_Sig20/1  "<testSig_CrCtl_vDesAct>"
  BS/21 -> ToWs_Req_Bus_Sig21/1  "<testSig_CrCtl_vDesActOld>"
  BS/22 -> ToWs_Req_Bus_Sig22/1  "<testSig_CrCtl_vMaxDvtAcc>"
  BS/23 -> ToWs_Req_Bus_Sig23/1  "<testSig_CrCtl_vMaxDvtDecl>"
  BS/24 -> ToWs_Req_Bus_Sig24/1  "<testSig_CrCtl_vMin>"
  BS/25 -> ToWs_Req_Bus_Sig25/1  "<testSig_EBrk_stPreSelMode>"
  BS/26 -> ToWs_Req_Bus_Sig26/1  "<testSig_EngDem_trqInrLim>"
  BS/27 -> ToWs_Req_Bus_Sig27/1  "<testSig_GlbDa_aXFlt>"
  BS/28 -> ToWs_Req_Bus_Sig28/1  "<testSig_GlbDa_vXFlt>"
  BS/29 -> ToWs_Req_Bus_Sig29/1  "<testSig_InjSys_trqLim>"
  BS/30 -> ToWs_Req_Bus_Sig30/1  "<testSig_PT_rTraV2N>"
  BS/31 -> ToWs_Req_Bus_Sig31/1  "<testSig_PT_rTrq>"
  BS/32 -> ToWs_Req_Bus_Sig32/1  "<testSig_PT_trqLos>"
  BS/33 -> ToWs_Req_Bus_Sig33/1  "<testSig_PT_trqWhl>"
  BS/34 -> ToWs_Req_Bus_Sig34/1  "<testSig_PT_trqWhlMinEng>"
  BS/35 -> ToWs_Req_Bus_Sig35/1  "<testSig_PT_trqWhlMinEngBrk>"
  BS/36 -> ToWs_Req_Bus_Sig36/1  "<testSig_RngMod_trqMin>"
  BS/37 -> ToWs_Req_Bus_Sig37/1  "<testSig_Tra_numGear>"
  BS/38 -> ToWs_Req_Bus_Sig38/1  "<testSig_VehMot_rTrqDfftl>"
  BS/39 -> ToWs_Req_Bus_Sig39/1  "<testSig_VMD_trqDes>"
  BS/40 -> ToWs_Req_Bus_Sig40/1  "<testSig_VMSAdjBtn_st>"
  BS/41 -> ToWs_Req_Bus_Sig41/1  "<testSig_VMSLmtSwt_st>"
  BS/42 -> ToWs_Req_Bus_Sig42/1  "<testSig_WESDem_stCurr>"
  BS/43 -> ToWs_Req_Bus_Sig43/1  "<testSig_CrCtl_rTraV2NBeg>"
  BS/44 -> ToWs_Req_Bus_Sig44/1  "<testSig_CrCtl_stOpFunc>"
  BS/45 -> ToWs_Req_Bus_Sig45/1  "<testSig_CrCtl_stPtd>"
  BS/46 -> ToWs_Req_Bus_Sig46/1  "<testSig_CrCtl_stReq>"
  BS/47 -> ToWs_Req_Bus_Sig47/1  "<testSig_CrCtl_stSuspRamp>"
  BS/48 -> ToWs_Req_Bus_Sig48/1  "<testSig_CrCtl_stvHysEngBrkReq>"
  BS/49 -> ToWs_Req_Bus_Sig49/1  "<testSig_CrCtl_trqLead>"
  BS/50 -> ToWs_Req_Bus_Sig50/1  "<testSig_CrCtl_trqLimAct>"
  BS/51 -> ToWs_Req_Bus_Sig51/1  "<testSig_CrCtl_trqMin>"
  BS/52 -> ToWs_Req_Bus_Sig52/1  "<testSig_CrCtl_trqReq>"
  BS/53 -> ToWs_Req_Bus_Sig53/1  "<testSig_CrCtl_trqReqOld>"
  BS/54 -> ToWs_Req_Bus_Sig54/1  "<testSig_CrCtl_vMax>"
  sig_Result_Bus/1 -> BS_Result/1, specifyOutputs/2(sig_Result_Bus)
  BS_Result/1 -> ToWs_Result_Bus_Sig1/1  "<CrCtl_rTraV2NBeg>"
  BS_Result/2 -> ToWs_Result_Bus_Sig2/1  "<CrCtl_stOpFunc>"
  BS_Result/3 -> ToWs_Result_Bus_Sig3/1  "<CrCtl_stPtd>"
  BS_Result/4 -> ToWs_Result_Bus_Sig4/1  "<CrCtl_stReq>"
  BS_Result/5 -> ToWs_Result_Bus_Sig5/1  "<CrCtl_stSuspRamp>"
  BS_Result/6 -> ToWs_Result_Bus_Sig6/1  "<CrCtl_stvHysEngBrkReq>"
  BS_Result/7 -> ToWs_Result_Bus_Sig7/1  "<CrCtl_trqLead>"
  BS_Result/8 -> ToWs_Result_Bus_Sig8/1  "<CrCtl_trqLimAct>"
  BS_Result/9 -> ToWs_Result_Bus_Sig9/1  "<CrCtl_trqMin>"
  BS_Result/10 -> ToWs_Result_Bus_Sig10/1  "<CrCtl_trqReq>"
  BS_Result/11 -> ToWs_Result_Bus_Sig11/1  "<CrCtl_trqReqOld>"
  BS_Result/12 -> ToWs_Result_Bus_Sig12/1  "<CrCtl_vMax>"
  specifyOutputs/1(result) -> result/1

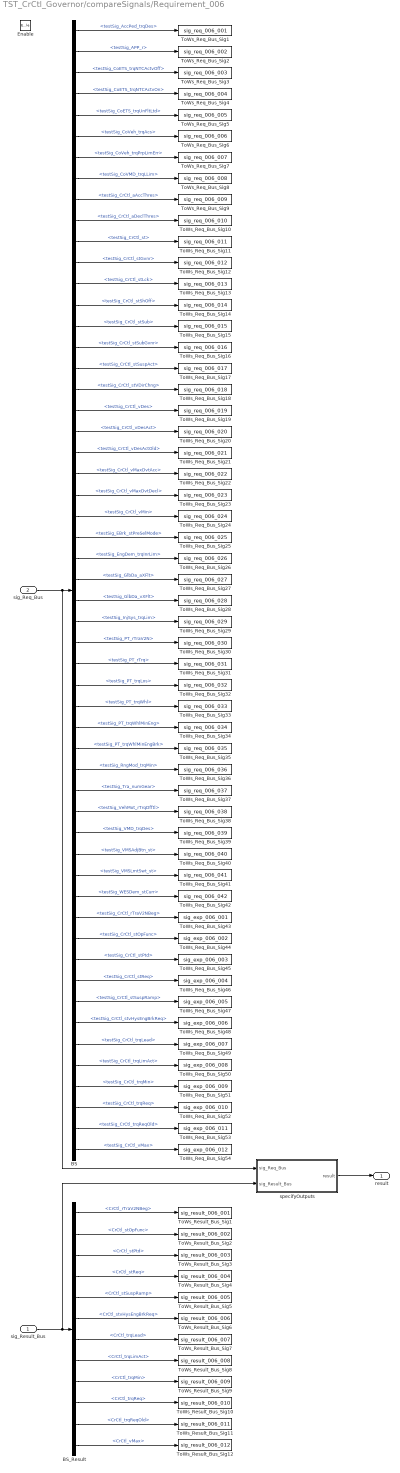
== system TST_CrCtl_Governor/compareSignals/Requirement_006 ==
  sig_Result_Bus : Inport
  sig_Req_Bus : Inport  Port=2
  Enable : EnablePort
  BS : BusSelector  OutputSignals=testSig_AccPed_trqDes,testSig_APP_r,testSig_CoETS_trqNTCActvOff,testSig_CoETS_trqNTCActvOn,testSig_CoETS_trqUnFltLtd,testSig_CoVeh_trqAcs,testSig_CoVeh_trqPrpLimErr,testSig_CoVMD_trqLLim,testSig_CrCtl_aAccThres,testSig_CrCtl_aDeclThres,testSig_CrCtl_st,testSig_CrCtl_stGvnr,testSig_CrCtl_stLck,testSig_CrCtl_stShOff,testSig_CrCtl_stSub,testSig_CrCtl_stSubGvnr,testSig_CrCtl_stSuspAct,testSig_CrCtl_stVDirChng,testSig_CrCtl_vDes,testSig_CrCtl_vDesAct,testSig_CrCtl_vDesActOld,testSig_CrCtl_vMaxDvtAcc,testSig_CrCtl_vMaxDvtDecl,testSig_CrCtl_vMin,testSig_EBrk_stPreSelMode,testSig_EngDem_trqInrLim,testSig_GlbDa_aXFlt,testSig_GlbDa_vXFlt,testSig_InjSys_trqLim,testSig_PT_rTraV2N,testSig_PT_rTrq,testSig_PT_trqLos,testSig_PT_trqWhl,testSig_PT_trqWhlMinEng,testSig_PT_trqWhlMinEngBrk,testSig_RngMod_trqMin,testSig_Tra_numGear,testSig_VehMot_rTrqDfftl,testSig_VMD_trqDes,testSig_VMSAdjBtn_st,testSig_VMSLmtSwt_st,testSig_WESDem_stCurr,testSig_CrCtl_rTraV2NBeg,testSig_CrCtl_stOpFunc,testSig_CrCtl_stPtd,testSig_CrCtl_stReq,testSig_CrCtl_stSuspRamp,testSig_CrCtl_stvHysEngBrkReq,testSig_CrCtl_trqLead,testSig_CrCtl_trqLimAct,testSig_CrCtl_trqMin,testSig_CrCtl_trqReq,testSig_CrCtl_trqReqOld,testSig_CrCtl_vMax
  BS_Result : BusSelector  OutputSignals=CrCtl_rTraV2NBeg,CrCtl_stOpFunc,CrCtl_stPtd,CrCtl_stReq,CrCtl_stSuspRamp,CrCtl_stvHysEngBrkReq,CrCtl_trqLead,CrCtl_trqLimAct,CrCtl_trqMin,CrCtl_trqReq,CrCtl_trqReqOld,CrCtl_vMax
  ToWs_Req_Bus_Sig1 : ToWorkspace  VariableName=sig_req_006_001  SaveFormat=Structure With Time
  ToWs_Req_Bus_Sig10 : ToWorkspace  VariableName=sig_req_006_010  SaveFormat=Structure With Time
  ToWs_Req_Bus_Sig11 : ToWorkspace  VariableName=sig_req_006_011  SaveFormat=Structure With Time
  ToWs_Req_Bus_Sig12 : ToWorkspace  VariableName=sig_req_006_012  SaveFormat=Structure With Time
  ToWs_Req_Bus_Sig13 : ToWorkspace  VariableName=sig_req_006_013  SaveFormat=Structure With Time
  ToWs_Req_Bus_Sig14 : ToWorkspace  VariableName=sig_req_006_014  SaveFormat=Structure With Time
  ToWs_Req_Bus_Sig15 : ToWorkspace  VariableName=sig_req_006_015  SaveFormat=Structure With Time
  ToWs_Req_Bus_Sig16 : ToWorkspace  VariableName=sig_req_006_016  SaveFormat=Structure With Time
  ToWs_Req_Bus_Sig17 : ToWorkspace  VariableName=sig_req_006_017  SaveFormat=Structure With Time
  ToWs_Req_Bus_Sig18 : ToWorkspace  VariableName=sig_req_006_018  SaveFormat=Structure With Time
  ToWs_Req_Bus_Sig19 : ToWorkspace  VariableName=sig_req_006_019  SaveFormat=Structure With Time
  ToWs_Req_Bus_Sig2 : ToWorkspace  VariableName=sig_req_006_002  SaveFormat=Structure With Time
  ToWs_Req_Bus_Sig20 : ToWorkspace  VariableName=sig_req_006_020  SaveFormat=Structure With Time
  ToWs_Req_Bus_Sig21 : ToWorkspace  VariableName=sig_req_006_021  SaveFormat=Structure With Time
  ToWs_Req_Bus_Sig22 : ToWorkspace  VariableName=sig_req_006_022  SaveFormat=Structure With Time
  ToWs_Req_Bus_Sig23 : ToWorkspace  VariableName=sig_req_006_023  SaveFormat=Structure With Time
  ToWs_Req_Bus_Sig24 : ToWorkspace  VariableName=sig_req_006_024  SaveFormat=Structure With Time
  ToWs_Req_Bus_Sig25 : ToWorkspace  VariableName=sig_req_006_025  SaveFormat=Structure With Time
  ToWs_Req_Bus_Sig26 : ToWorkspace  VariableName=sig_req_006_026  SaveFormat=Structure With Time
  ToWs_Req_Bus_Sig27 : ToWorkspace  VariableName=sig_req_006_027  SaveFormat=Structure With Time
  ToWs_Req_Bus_Sig28 : ToWorkspace  VariableName=sig_req_006_028  SaveFormat=Structure With Time
  ToWs_Req_Bus_Sig29 : ToWorkspace  VariableName=sig_req_006_029  SaveFormat=Structure With Time
  ToWs_Req_Bus_Sig3 : ToWorkspace  VariableName=sig_req_006_003  SaveFormat=Structure With Time
  ToWs_Req_Bus_Sig30 : ToWorkspace  VariableName=sig_req_006_030  SaveFormat=Structure With Time
  ToWs_Req_Bus_Sig31 : ToWorkspace  VariableName=sig_req_006_031  SaveFormat=Structure With Time
  ToWs_Req_Bus_Sig32 : ToWorkspace  VariableName=sig_req_006_032  SaveFormat=Structure With Time
  ToWs_Req_Bus_Sig33 : ToWorkspace  VariableName=sig_req_006_033  SaveFormat=Structure With Time
  ToWs_Req_Bus_Sig34 : ToWorkspace  VariableName=sig_req_006_034  SaveFormat=Structure With Time
  ToWs_Req_Bus_Sig35 : ToWorkspace  VariableName=sig_req_006_035  SaveFormat=Structure With Time
  ToWs_Req_Bus_Sig36 : ToWorkspace  VariableName=sig_req_006_036  SaveFormat=Structure With Time
  ToWs_Req_Bus_Sig37 : ToWorkspace  VariableName=sig_req_006_037  SaveFormat=Structure With Time
  ToWs_Req_Bus_Sig38 : ToWorkspace  VariableName=sig_req_006_038  SaveFormat=Structure With Time
  ToWs_Req_Bus_Sig39 : ToWorkspace  VariableName=sig_req_006_039  SaveFormat=Structure With Time
  ToWs_Req_Bus_Sig4 : ToWorkspace  VariableName=sig_req_006_004  SaveFormat=Structure With Time
  ToWs_Req_Bus_Sig40 : ToWorkspace  VariableName=sig_req_006_040  SaveFormat=Structure With Time
  ToWs_Req_Bus_Sig41 : ToWorkspace  VariableName=sig_req_006_041  SaveFormat=Structure With Time
  ToWs_Req_Bus_Sig42 : ToWorkspace  VariableName=sig_req_006_042  SaveFormat=Structure With Time
  ToWs_Req_Bus_Sig43 : ToWorkspace  VariableName=sig_exp_006_001  SaveFormat=Structure With Time
  ToWs_Req_Bus_Sig44 : ToWorkspace  VariableName=sig_exp_006_002  SaveFormat=Structure With Time
  ToWs_Req_Bus_Sig45 : ToWorkspace  VariableName=sig_exp_006_003  SaveFormat=Structure With Time
  ToWs_Req_Bus_Sig46 : ToWorkspace  VariableName=sig_exp_006_004  SaveFormat=Structure With Time
  ToWs_Req_Bus_Sig47 : ToWorkspace  VariableName=sig_exp_006_005  SaveFormat=Structure With Time
  ToWs_Req_Bus_Sig48 : ToWorkspace  VariableName=sig_exp_006_006  SaveFormat=Structure With Time
  ToWs_Req_Bus_Sig49 : ToWorkspace  VariableName=sig_exp_006_007  SaveFormat=Structure With Time
  ToWs_Req_Bus_Sig5 : ToWorkspace  VariableName=sig_req_006_005  SaveFormat=Structure With Time
  ToWs_Req_Bus_Sig50 : ToWorkspace  VariableName=sig_exp_006_008  SaveFormat=Structure With Time
  ToWs_Req_Bus_Sig51 : ToWorkspace  VariableName=sig_exp_006_009  SaveFormat=Structure With Time
  ToWs_Req_Bus_Sig52 : ToWorkspace  VariableName=sig_exp_006_010  SaveFormat=Structure With Time
  ToWs_Req_Bus_Sig53 : ToWorkspace  VariableName=sig_exp_006_011  SaveFormat=Structure With Time
  ToWs_Req_Bus_Sig54 : ToWorkspace  VariableName=sig_exp_006_012  SaveFormat=Structure With Time
  ToWs_Req_Bus_Sig6 : ToWorkspace  VariableName=sig_req_006_006  SaveFormat=Structure With Time
  ToWs_Req_Bus_Sig7 : ToWorkspace  VariableName=sig_req_006_007  SaveFormat=Structure With Time
  ToWs_Req_Bus_Sig8 : ToWorkspace  VariableName=sig_req_006_008  SaveFormat=Structure With Time
  ToWs_Req_Bus_Sig9 : ToWorkspace  VariableName=sig_req_006_009  SaveFormat=Structure With Time
  ToWs_Result_Bus_Sig1 : ToWorkspace  VariableName=sig_result_006_001  SaveFormat=Structure With Time
  ToWs_Result_Bus_Sig10 : ToWorkspace  VariableName=sig_result_006_010  SaveFormat=Structure With Time
  ToWs_Result_Bus_Sig11 : ToWorkspace  VariableName=sig_result_006_011  SaveFormat=Structure With Time
  ToWs_Result_Bus_Sig12 : ToWorkspace  VariableName=sig_result_006_012  SaveFormat=Structure With Time
  ToWs_Result_Bus_Sig2 : ToWorkspace  VariableName=sig_result_006_002  SaveFormat=Structure With Time
  ToWs_Result_Bus_Sig3 : ToWorkspace  VariableName=sig_result_006_003  SaveFormat=Structure With Time
  ToWs_Result_Bus_Sig4 : ToWorkspace  VariableName=sig_result_006_004  SaveFormat=Structure With Time
  ToWs_Result_Bus_Sig5 : ToWorkspace  VariableName=sig_result_006_005  SaveFormat=Structure With Time
  ToWs_Result_Bus_Sig6 : ToWorkspace  VariableName=sig_result_006_006  SaveFormat=Structure With Time
  ToWs_Result_Bus_Sig7 : ToWorkspace  VariableName=sig_result_006_007  SaveFormat=Structure With Time
  ToWs_Result_Bus_Sig8 : ToWorkspace  VariableName=sig_result_006_008  SaveFormat=Structure With Time
  ToWs_Result_Bus_Sig9 : ToWorkspace  VariableName=sig_result_006_009  SaveFormat=Structure With Time
  specifyOutputs : Subsystem
  result : Outport
  wires:
  sig_Req_Bus/1 -> BS/1, specifyOutputs/1(sig_Req_Bus)
  BS/1 -> ToWs_Req_Bus_Sig1/1  "<testSig_AccPed_trqDes>"
  BS/2 -> ToWs_Req_Bus_Sig2/1  "<testSig_APP_r>"
  BS/3 -> ToWs_Req_Bus_Sig3/1  "<testSig_CoETS_trqNTCActvOff>"
  BS/4 -> ToWs_Req_Bus_Sig4/1  "<testSig_CoETS_trqNTCActvOn>"
  BS/5 -> ToWs_Req_Bus_Sig5/1  "<testSig_CoETS_trqUnFltLtd>"
  BS/6 -> ToWs_Req_Bus_Sig6/1  "<testSig_CoVeh_trqAcs>"
  BS/7 -> ToWs_Req_Bus_Sig7/1  "<testSig_CoVeh_trqPrpLimErr>"
  BS/8 -> ToWs_Req_Bus_Sig8/1  "<testSig_CoVMD_trqLLim>"
  BS/9 -> ToWs_Req_Bus_Sig9/1  "<testSig_CrCtl_aAccThres>"
  BS/10 -> ToWs_Req_Bus_Sig10/1  "<testSig_CrCtl_aDeclThres>"
  BS/11 -> ToWs_Req_Bus_Sig11/1  "<testSig_CrCtl_st>"
  BS/12 -> ToWs_Req_Bus_Sig12/1  "<testSig_CrCtl_stGvnr>"
  BS/13 -> ToWs_Req_Bus_Sig13/1  "<testSig_CrCtl_stLck>"
  BS/14 -> ToWs_Req_Bus_Sig14/1  "<testSig_CrCtl_stShOff>"
  BS/15 -> ToWs_Req_Bus_Sig15/1  "<testSig_CrCtl_stSub>"
  BS/16 -> ToWs_Req_Bus_Sig16/1  "<testSig_CrCtl_stSubGvnr>"
  BS/17 -> ToWs_Req_Bus_Sig17/1  "<testSig_CrCtl_stSuspAct>"
  BS/18 -> ToWs_Req_Bus_Sig18/1  "<testSig_CrCtl_stVDirChng>"
  BS/19 -> ToWs_Req_Bus_Sig19/1  "<testSig_CrCtl_vDes>"
  BS/20 -> ToWs_Req_Bus_Sig20/1  "<testSig_CrCtl_vDesAct>"
  BS/21 -> ToWs_Req_Bus_Sig21/1  "<testSig_CrCtl_vDesActOld>"
  BS/22 -> ToWs_Req_Bus_Sig22/1  "<testSig_CrCtl_vMaxDvtAcc>"
  BS/23 -> ToWs_Req_Bus_Sig23/1  "<testSig_CrCtl_vMaxDvtDecl>"
  BS/24 -> ToWs_Req_Bus_Sig24/1  "<testSig_CrCtl_vMin>"
  BS/25 -> ToWs_Req_Bus_Sig25/1  "<testSig_EBrk_stPreSelMode>"
  BS/26 -> ToWs_Req_Bus_Sig26/1  "<testSig_EngDem_trqInrLim>"
  BS/27 -> ToWs_Req_Bus_Sig27/1  "<testSig_GlbDa_aXFlt>"
  BS/28 -> ToWs_Req_Bus_Sig28/1  "<testSig_GlbDa_vXFlt>"
  BS/29 -> ToWs_Req_Bus_Sig29/1  "<testSig_InjSys_trqLim>"
  BS/30 -> ToWs_Req_Bus_Sig30/1  "<testSig_PT_rTraV2N>"
  BS/31 -> ToWs_Req_Bus_Sig31/1  "<testSig_PT_rTrq>"
  BS/32 -> ToWs_Req_Bus_Sig32/1  "<testSig_PT_trqLos>"
  BS/33 -> ToWs_Req_Bus_Sig33/1  "<testSig_PT_trqWhl>"
  BS/34 -> ToWs_Req_Bus_Sig34/1  "<testSig_PT_trqWhlMinEng>"
  BS/35 -> ToWs_Req_Bus_Sig35/1  "<testSig_PT_trqWhlMinEngBrk>"
  BS/36 -> ToWs_Req_Bus_Sig36/1  "<testSig_RngMod_trqMin>"
  BS/37 -> ToWs_Req_Bus_Sig37/1  "<testSig_Tra_numGear>"
  BS/38 -> ToWs_Req_Bus_Sig38/1  "<testSig_VehMot_rTrqDfftl>"
  BS/39 -> ToWs_Req_Bus_Sig39/1  "<testSig_VMD_trqDes>"
  BS/40 -> ToWs_Req_Bus_Sig40/1  "<testSig_VMSAdjBtn_st>"
  BS/41 -> ToWs_Req_Bus_Sig41/1  "<testSig_VMSLmtSwt_st>"
  BS/42 -> ToWs_Req_Bus_Sig42/1  "<testSig_WESDem_stCurr>"
  BS/43 -> ToWs_Req_Bus_Sig43/1  "<testSig_CrCtl_rTraV2NBeg>"
  BS/44 -> ToWs_Req_Bus_Sig44/1  "<testSig_CrCtl_stOpFunc>"
  BS/45 -> ToWs_Req_Bus_Sig45/1  "<testSig_CrCtl_stPtd>"
  BS/46 -> ToWs_Req_Bus_Sig46/1  "<testSig_CrCtl_stReq>"
  BS/47 -> ToWs_Req_Bus_Sig47/1  "<testSig_CrCtl_stSuspRamp>"
  BS/48 -> ToWs_Req_Bus_Sig48/1  "<testSig_CrCtl_stvHysEngBrkReq>"
  BS/49 -> ToWs_Req_Bus_Sig49/1  "<testSig_CrCtl_trqLead>"
  BS/50 -> ToWs_Req_Bus_Sig50/1  "<testSig_CrCtl_trqLimAct>"
  BS/51 -> ToWs_Req_Bus_Sig51/1  "<testSig_CrCtl_trqMin>"
  BS/52 -> ToWs_Req_Bus_Sig52/1  "<testSig_CrCtl_trqReq>"
  BS/53 -> ToWs_Req_Bus_Sig53/1  "<testSig_CrCtl_trqReqOld>"
  BS/54 -> ToWs_Req_Bus_Sig54/1  "<testSig_CrCtl_vMax>"
  sig_Result_Bus/1 -> BS_Result/1, specifyOutputs/2(sig_Result_Bus)
  BS_Result/1 -> ToWs_Result_Bus_Sig1/1  "<CrCtl_rTraV2NBeg>"
  BS_Result/2 -> ToWs_Result_Bus_Sig2/1  "<CrCtl_stOpFunc>"
  BS_Result/3 -> ToWs_Result_Bus_Sig3/1  "<CrCtl_stPtd>"
  BS_Result/4 -> ToWs_Result_Bus_Sig4/1  "<CrCtl_stReq>"
  BS_Result/5 -> ToWs_Result_Bus_Sig5/1  "<CrCtl_stSuspRamp>"
  BS_Result/6 -> ToWs_Result_Bus_Sig6/1  "<CrCtl_stvHysEngBrkReq>"
  BS_Result/7 -> ToWs_Result_Bus_Sig7/1  "<CrCtl_trqLead>"
  BS_Result/8 -> ToWs_Result_Bus_Sig8/1  "<CrCtl_trqLimAct>"
  BS_Result/9 -> ToWs_Result_Bus_Sig9/1  "<CrCtl_trqMin>"
  BS_Result/10 -> ToWs_Result_Bus_Sig10/1  "<CrCtl_trqReq>"
  BS_Result/11 -> ToWs_Result_Bus_Sig11/1  "<CrCtl_trqReqOld>"
  BS_Result/12 -> ToWs_Result_Bus_Sig12/1  "<CrCtl_vMax>"
  specifyOutputs/1(result) -> result/1
